simulink model "dus4"  (R2014a)
settings: Solver=FixedStepDiscrete  StartTime=0.0  StopTime=10.0  FixedStep=0.1  RelTol=1e-3
settings Model: Creator=yoshi12  LastModifiedBy=yoshi12

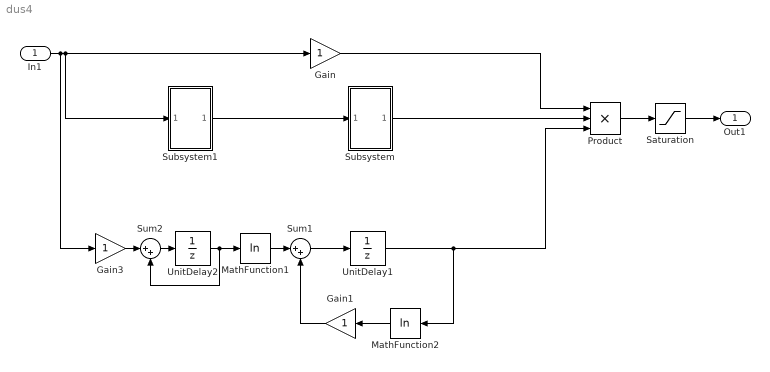
== system dus4 ==
  In1 : Inport
  Gain : Gain
  Gain1 : Gain
  Gain3 : Gain
  MathFunction1 : Math  Operator=log  SaturateOnIntegerOverflow=on
  MathFunction2 : Math  Operator=log  SaturateOnIntegerOverflow=on
  Product : Product  Inputs=3
  Saturation : Saturate
  Subsystem : Subsystem
  Subsystem1 : Subsystem
  Sum1 : Sum  Inputs=|++
  Sum2 : Sum  Inputs=|++
  UnitDelay1 : UnitDelay  SampleTime=-1
  UnitDelay2 : UnitDelay  SampleTime=-1
  Out1 : Outport
  wires:
  In1/1 -> Gain3/1, Subsystem1/1(In1), Gain/1
  Gain/1 -> Product/1
  Product/1 -> Saturation/1
  Saturation/1 -> Out1/1
  Gain3/1 -> Sum2/1
  MathFunction1/1 -> Sum1/1
  UnitDelay1/1 -> MathFunction2/1, Product/3
  Sum1/1 -> UnitDelay1/1
  Subsystem/1(Out1) -> Product/2
  Subsystem1/1(Out1) -> Subsystem/1(In1)
  UnitDelay2/1 -> MathFunction1/1, Sum2/2
  Sum2/1 -> UnitDelay2/1
  Gain1/1 -> Sum1/2
  MathFunction2/1 -> Gain1/1

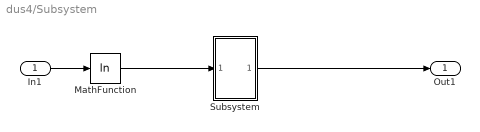
== system dus4/Subsystem ==
  In1 : Inport
  MathFunction : Math  Operator=log  SaturateOnIntegerOverflow=on
  Subsystem : Subsystem
  Out1 : Outport
  wires:
  In1/1 -> MathFunction/1
  MathFunction/1 -> Subsystem/1(In1)
  Subsystem/1(Out1) -> Out1/1

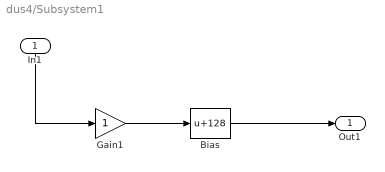
== system dus4/Subsystem1 ==
  In1 : Inport
  Bias : Bias  Bias=128
  Gain1 : Gain
  Out1 : Outport
  wires:
  Gain1/1 -> Bias/1
  Bias/1 -> Out1/1
  In1/1 -> Gain1/1

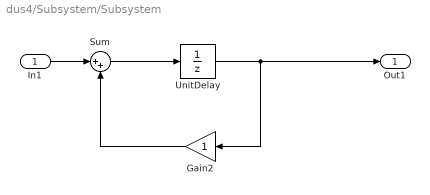
== system dus4/Subsystem/Subsystem ==
  In1 : Inport
  Gain2 : Gain
  Sum : Sum  Inputs=|++
  UnitDelay : UnitDelay  SampleTime=-1
  Out1 : Outport
  wires:
  Sum/1 -> UnitDelay/1
  UnitDelay/1 -> Out1/1, Gain2/1
  In1/1 -> Sum/1
  Gain2/1 -> Sum/2
